simulink model "levitador_mpc_ss_du"  (Simulink 7.9)
settings: Solver=ode5  SolverMode=SingleTasking  StartTime=0.0  StopTime=2  FixedStep=0.001  RelTol=1e-3
values from neighbouring files (symbols this model uses):
  C = [1 0]    [parametros_maglev_ss.m]
  dend = [1 0]    [parametros_maglev_ss.m]
  g = 9.8    [parametros_maglev_ss.m]
  gamma = 328    [parametros_maglev_ss.m]
  i0 = 0.514    [parametros_maglev_ss.m]
  Kf = 1.2e-4    (= 0.00012)    [parametros_maglev_ss.m]
  KMPC = aux2(1,:)    [matrizes_ss_du.m]
  mass = 2.12e-2    (= 0.0212)    [parametros_maglev_ss.m]
  numd = [1/T -1/T]    [parametros_maglev_ss.m]
  r = 0.166    [parametros_maglev_ss.m]
  T = 0.005    [parametros_maglev_ss.m]
  up_equilibrio = ( sqrt(mass*g/Kf)*(yp_equilibrio - y0) / gamma - i0 ) / r    [parametros_maglev_ss.m]
  y0 = -7.47    [parametros_maglev_ss.m]
  yp_equilibrio = 0    [parametros_maglev_ss.m]
undefined symbols (not defined in the file or in its folder): A, B, Phi
settings Model: Creator=Kawakami  LastModifiedBy=Kawakami
settings DataIOCC: SignalLoggingName=sigsOut
settings OptimizationCC: BooleanDataType=off
settings DebuggingCC: SaveWithParameterizedLinksMsg=none  SignalResolutionControl=TryResolveAllWithWarning  SolverPrmCheckMsg=none  MultiTaskDSMMsg=warning  MultiTaskCondExecSysMsg=none  FcnCallInpInsideContextMsg=Use local settings  StrictBusMsg=None
settings HardwareCC: TargetUnknown=on
settings RTWCC: IncludeERTFirstTime=on
settings GRTTargetCC: CombineOutputUpdateFcns=off  GRTInterface=on

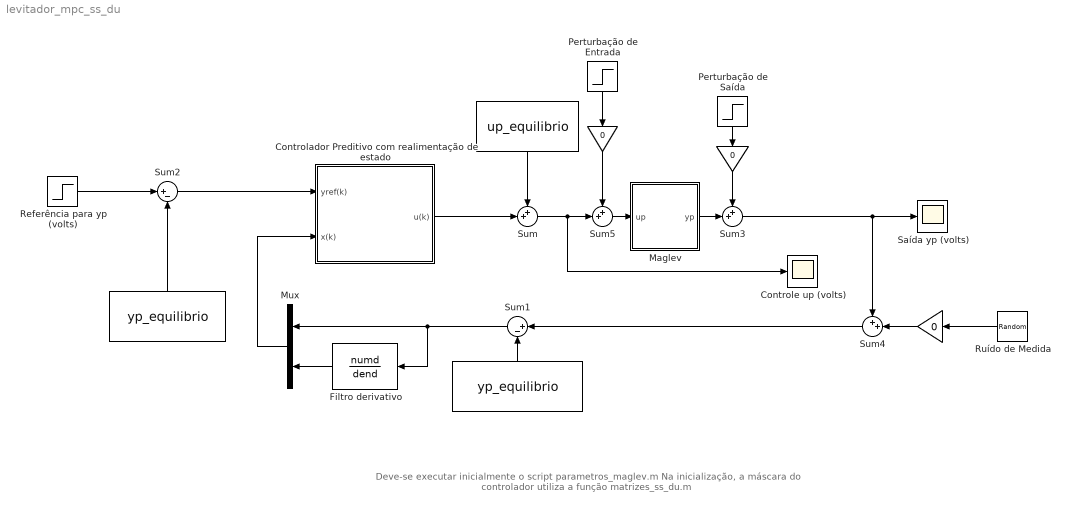
== system levitador_mpc_ss_du ==
  note: Deve-se executar inicialmente o script parametros_maglev.m
      |
      | Na inicialização, a máscara do controlador utiliza a função matrizes_ss_du.m
  " " : Constant  Value=yp_equilibrio
  "  " : Constant  Value=yp_equilibrio
  "   " : Constant  Value=up_equilibrio
  "    " : Gain  Gain=0
  "     " : Gain  Gain=0
  "      " : Gain  Gain=0
  Controlador Preditivo com realimentação de estado : Subsystem  mask{rho=1, N=20, M=5, A=A, B=B, C=C, T=T}
      mask prompts: rho "Peso do controle (rho)"; N "Horizonte de Predição (N)"; M "Horizonte de Controle (M)"; A "Matriz A"; B "Matriz B"; C "Matriz C"; T "Periodo de amostragem"
      mask init:
      | [KMPC,Phi] = matrizes_ss_du(A,B,C,N,M,rho);
  Controle up (volts) : Scope
      settings: TimeRange=2  YMin=2  YMax=3.5  SaveName=y1
  Filtro derivativo : DiscreteTransferFcn  Numerator=numd  Denominator=dend  SampleTime=T
  Maglev : Subsystem  mask{mass=mass, g=g, y0=y0, gamma=gamma, i0=i0, r=r, Kf=Kf, yp_inicial=yp_equilibrio, T=T}
      mask prompts: mass "massa (kg)"; g "g (m/s^2)"; y0 "y0 (V)"; gamma "gamma (V/m)"; i0 "i0 (A)"; r "r (A/V)"; Kf "Kf (N*m^2/A^2)"; yp_inicial "yp inicial (V)"; T "Periodo de Amostragem (s)"
  Mux : Mux  Inputs=2
  Perturbação de Entrada : Step  After=0.5  SampleTime=0
  Perturbação de Saída : Step  After=0.2  SampleTime=0
  Referência para yp (volts) : Step  Time=0.2  After=0.5  SampleTime=0
  Ruído de Medida : RandomNumber  Variance=0.0001  SampleTime=T
  Saída yp (volts) : Scope
      settings: TimeRange=2  YMin=0  YMax=0.7000000000000001  SaveName=y
  Sum{,3..5} (4 alike) : Sum  Inputs=++|  SaturateOnIntegerOverflow=on
  Sum1 : Sum  Inputs=|+-  SaturateOnIntegerOverflow=on
  Sum2 : Sum  Inputs=|+-  SaturateOnIntegerOverflow=on
  wires:
  Controlador Preditivo com realimentação de estado/1(u(k)) -> Sum/2
  Sum2/1 -> Controlador Preditivo com realimentação de estado/1(yref(k))
  Referência para yp (volts)/1 -> Sum2/1
  Maglev/1(yp) -> Sum3/2
  Sum3/1 -> Saída yp (volts)/1, Sum4/1
  Sum4/1 -> Sum1/1
  Perturbação de Saída/1 -> "     "/1
  Sum/1 -> Sum5/2, Controle up (volts)/1
  Sum5/1 -> Maglev/1(up)
  Perturbação de Entrada/1 -> "    "/1
  Ruído de Medida/1 -> "      "/1
  Sum1/1 -> Mux/1, Filtro derivativo/1
  Mux/1 -> Controlador Preditivo com realimentação de estado/2(x(k))
  "  "/1 -> Sum2/2
  "   "/1 -> Sum/1
  " "/1 -> Sum1/2
  Filtro derivativo/1 -> Mux/2
  "    "/1 -> Sum5/1
  "     "/1 -> Sum3/1
  "      "/1 -> Sum4/2

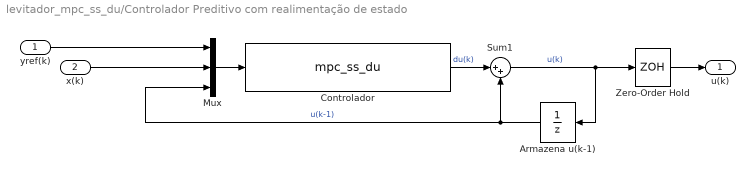
== system levitador_mpc_ss_du/Controlador Preditivo com realimentação de estado ==
  yref(k) : Inport
  x(k) : Inport  Port=2
  Armazena u(k-1) : UnitDelay  SampleTime=T
  Controlador : S-Function  FunctionName=mpc_ss_du  Parameters=KMPC,Phi,T  EnableBusSupport=off
  Mux : Mux  Inputs=3
  Sum1 : Sum  Inputs=|++  SaturateOnIntegerOverflow=on  InputSameDT=on  OutDataTypeStr=Inherit: Same as first input
  Zero-Order Hold : ZeroOrderHold  SampleTime=T
  u(k) : Outport
  wires:
  Mux/1 -> Controlador/1
  Zero-Order Hold/1 -> u(k)/1
  x(k)/1 -> Mux/2
  yref(k)/1 -> Mux/1
  Sum1/1 -> Zero-Order Hold/1, Armazena u(k-1)/1  "u(k)"
  Armazena u(k-1)/1 -> Sum1/2, Mux/3  "u(k-1)"
  Controlador/1 -> Sum1/1  "du(k)"

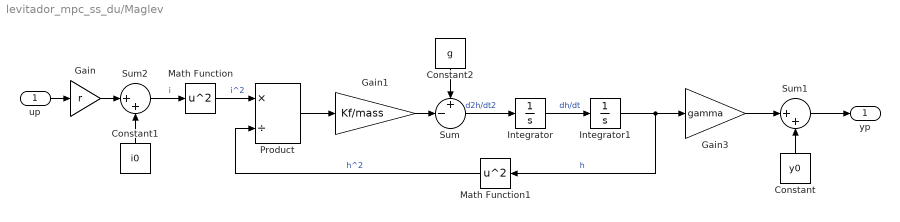
== system levitador_mpc_ss_du/Maglev ==
  up : Inport
  Constant : Constant  Value=y0
  Constant1 : Constant  Value=i0
  Constant2 : Constant  Value=g
  Gain : Gain  Gain=r  SaturateOnIntegerOverflow=on  OutDataTypeStr=Inherit: Same as input  ParamDataTypeStr=Inherit: Same as input
  Gain1 : Gain  Gain=Kf/mass  SaturateOnIntegerOverflow=on  OutDataTypeStr=Inherit: Same as input  ParamDataTypeStr=Inherit: Same as input
  Gain3 : Gain  Gain=gamma  SaturateOnIntegerOverflow=on  OutDataTypeStr=Inherit: Same as input  ParamDataTypeStr=Inherit: Same as input
  Integrator : Integrator
  Integrator1 : Integrator  InitialCondition=(yp_inicial - y0)/gamma
  Math Function : Math  Operator=square  SaturateOnIntegerOverflow=on
  Math Function1 : Math  Operator=square  SaturateOnIntegerOverflow=on
  Product : Product  Inputs=*/  SaturateOnIntegerOverflow=on  OutDataTypeStr=Inherit: Same as first input
  Sum : Sum  Inputs=+-|  SaturateOnIntegerOverflow=on
  Sum1 : Sum  Inputs=|++  SaturateOnIntegerOverflow=on
  Sum2 : Sum  Inputs=|++  SaturateOnIntegerOverflow=on
  yp : Outport
  wires:
  Integrator/1 -> Integrator1/1  "dh/dt"
  Sum/1 -> Integrator/1  "d2h/dt2"
  Integrator1/1 -> Gain3/1, Math Function1/1  "h"
  up/1 -> Gain/1
  Constant/1 -> Sum1/2
  Gain3/1 -> Sum1/1
  Sum1/1 -> yp/1
  Constant1/1 -> Sum2/2
  Gain/1 -> Sum2/1
  Sum2/1 -> Math Function/1  "i"
  Math Function/1 -> Product/1  "i^2"
  Math Function1/1 -> Product/2  "h^2"
  Product/1 -> Gain1/1
  Gain1/1 -> Sum/2
  Constant2/1 -> Sum/1
